simulink model "Q_3_2_a"  (R2023b)
settings: Solver=VariableStepAuto  StartTime=0.0  StopTime=400e-3  MaxStep=tstepMax  RelTol=1e-3
values from neighbouring files (symbols this model uses):
  v_in = 15*sqrt(2)    [Q3_2.m]    (also in thyristor.m = 20)
libraries: spsDiodeLib x6, spsSeriesRLCBranchLib x4, spsACVoltageSourceLib x3, spsCurrentMeasurementLib x2, spsVoltageMeasurementLib x2, spsControlledCurrentSourceLib x1, spsControlledVoltageSourceLib x1, spspowerguiLib x1
settings Model: Creator=abdulkadir  LastModifiedBy=abdulkadir
settings DataIOCC: ReturnWorkspaceOutputs=off

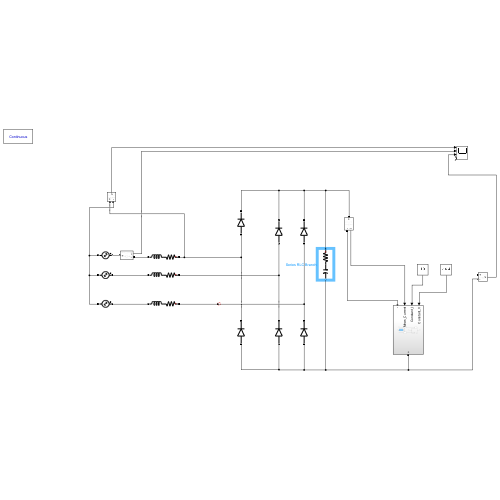
[thumbnail: Simulink's stored preview of the top-level diagram]
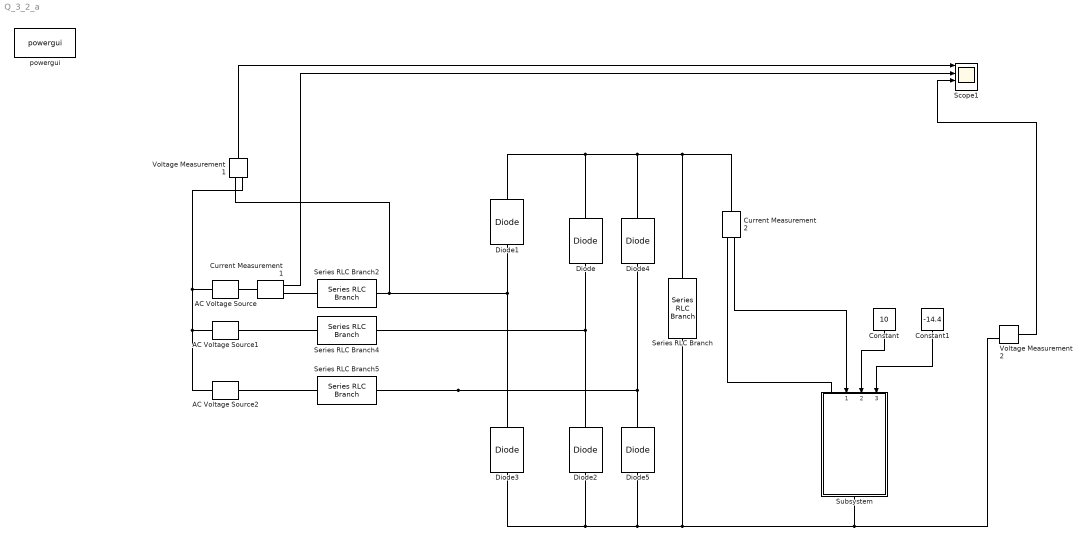
== system Q_3_2_a ==
  AC Voltage Source : spsACVoltageSourceLib/AC Voltage Source  Amplitude=v_in  Phase=0  Frequency=50  SampleTime=0  Measurements=None  BusType=swing  Pref=10e3  Qref=0  Qmin=-inf  Qmax=+inf
  AC Voltage Source1 : spsACVoltageSourceLib/AC Voltage Source  Amplitude=v_in  Phase=120  Frequency=50  SampleTime=0  Measurements=None  BusType=swing  Pref=10e3  Qref=0  Qmin=-inf  Qmax=+inf
  AC Voltage Source2 : spsACVoltageSourceLib/AC Voltage Source  Amplitude=v_in  Phase=240  Frequency=50  SampleTime=0  Measurements=None  BusType=swing  Pref=10e3  Qref=0  Qmin=-inf  Qmax=+inf
  Constant : Constant  Value=10
  Constant1 : Constant  Value=-14.4
  Current Measurement1 : spsCurrentMeasurementLib/Current Measurement  PhasorSimulation=off  OutputType=Complex  PSBequivalent=0
  Current Measurement2 : spsCurrentMeasurementLib/Current Measurement  PhasorSimulation=off  OutputType=Complex  PSBequivalent=0
  Diode{,1..5} (6 alike) : spsDiodeLib/Diode  Ron=0  Lon=0  Vf=0  IC=0  UseSnubber=0  Rs=0  Cs=0  Measurements=off
  Scope1 : Scope  NumInputPorts=4
  Series RLC Branch : spsSeriesRLCBranchLib/Series RLC Branch  LConnTagsString=__new0  RConnTagsString=__new0  BranchType=RC  Resistance=1e-3  Inductance=1e-3  SetiL0=off  InitialCurrent=0  Capacitance=470e-6  Setx0=off  InitialVoltage=0  Measurements=None
  Series RLC Branch2 : spsSeriesRLCBranchLib/Series RLC Branch  LConnTagsString=__new0  RConnTagsString=__new0  BranchType=RL  Resistance=0.05  Inductance=0.28e-3  SetiL0=off  InitialCurrent=0  Capacitance=470e-6  Setx0=off  InitialVoltage=0  Measurements=None
  Series RLC Branch4 : spsSeriesRLCBranchLib/Series RLC Branch  LConnTagsString=__new0  RConnTagsString=__new0  BranchType=RL  Resistance=0.1  Inductance=0.28e-3  SetiL0=off  InitialCurrent=0  Capacitance=470e-6  Setx0=off  InitialVoltage=0  Measurements=None
  Series RLC Branch5 : spsSeriesRLCBranchLib/Series RLC Branch  LConnTagsString=__new0  RConnTagsString=__new0  BranchType=RL  Resistance=0.1  Inductance=0.28e-3  SetiL0=off  InitialCurrent=0  Capacitance=470e-6  Setx0=off  InitialVoltage=0  Measurements=None
  Subsystem : Subsystem
      settings: PortSchema="{\"entries\":[{\"content\":{\"sides\":[{\"content\":{\"connectorIds\":[\"LConn1\",\"In1\",\"In2\",\"In3\"]},\"type\":\"ConnectorPlacement.EquallySpacedRectSide\",\"uuid\":\"feaae4e9-bb6a-4e16-aae7-51a0d38361ce\"},{\"content\":{\"connectorIds\":[\"RConn1\"],\"side\":\"RIGHT\"},\"type\":\"ConnectorPlacement.EquallySpacedRectSide\",\"uuid\":\"0242307e-3fb3-4380-a5a2-342063310801\"},{\"content\":{\"side\":\"TOP\"},\"type\":\"ConnectorPlacement.EquallySpacedRectSide\",\"uuid\":\"eff0ed2a-871e-41c2-ba24-befc3dd8f64b\"}]},\"type\":\"ConnectorPlacement.EquallySpacedConnector\",\"uuid\":\"58606344-83d6-409b-9606-3c46dbcf5736\"}],\"packageUris\":[\"http://schema.mathworks.com/mf0/Connector/R2020b\"],\"version\":\"1.0\"}"
  Voltage Measurement1 : spsVoltageMeasurementLib/Voltage Measurement  PhasorSimulation=off  OutputType=Complex  PSBequivalent=0
  Voltage Measurement2 : spsVoltageMeasurementLib/Voltage Measurement  PhasorSimulation=off  OutputType=Complex  PSBequivalent=0
  powergui : spspowerguiLib/powergui  Priority=1  SimulationMode=Continuous  SampleTime=0.1e-3  frequency=60  Iterations=50  frequencyindice=50  Pbase=100e6  ErrMax=1e-4  UnitsV=kV  UnitsW=MW  buscounter=0  FunctionMessages=off  echomessages=off  EnableUseOfTLC=off  CurrentSourceSwitches=off  DisableSnubberDevices=off  DisableRonSwitches=off  DisableVfSwitches=off  DisplayEquations=off  AutomaticDiscreteSolvers=off  SolverType=Tustin/Backward Euler (TBE)  Interpol=off  ExternalGateDelay=off  methode=off  Ts=100  x0status=blocks  SPID=on  SwTol=0  HookPort=off  NonlinearTolerance=1e-4  nMaxIteration=100  ContinueOnMaxIteration=off  RestoreLinks=warning  ResistiveCurrentMeasurement=off  Frange=[0:2:500]  Ylog=off  Xlog=on  ShowGrid=off  save=off  variable=ZData  structure=0  ZoomFFT=off  StartTime=0.0  cycles=1  DisplayStyle=1  fundamental=60  FreqAxis=off  MaxFrequency=1000  frequencyindicesteady=1  RmsSteady=1  display=off
  wires:
  Current Measurement1/1 -> Scope1/2
  Voltage Measurement2/1 -> Scope1/3
  Voltage Measurement1/1 -> Scope1/1
  Current Measurement2/1 -> Subsystem/1(Meas_Current)
  Constant/1 -> Subsystem/2(Constant_I)
  Constant1/1 -> Subsystem/3(Constant_V)
  connections:
  Series RLC Branch/LConn1 -- Diode4/RConn1 -- Diode1/RConn1 -- Diode/RConn1 -- Current Measurement2/LConn1
  Series RLC Branch/RConn1 -- Subsystem/RConn1 -- Voltage Measurement2/LConn2 -- Diode5/LConn1 -- Diode3/LConn1 -- Diode2/LConn1
  Current Measurement1/LConn1 -- AC Voltage Source/RConn1
  Series RLC Branch2/LConn1 -- Diode1/LConn1 -- Diode3/RConn1 -- Voltage Measurement1/LConn1
  Current Measurement1/RConn1 -- Series RLC Branch2/RConn1
  Series RLC Branch4/RConn1 -- AC Voltage Source1/RConn1
  Series RLC Branch5/RConn1 -- AC Voltage Source2/RConn1
  Diode2/RConn1 -- Series RLC Branch4/LConn1 -- Diode/LConn1
  Voltage Measurement1/LConn2 -- AC Voltage Source/LConn1 -- AC Voltage Source2/LConn1 -- AC Voltage Source1/LConn1
  Diode5/RConn1 -- Series RLC Branch5/LConn1 -- Diode4/LConn1
  Subsystem/LConn1 -- Current Measurement2/RConn1

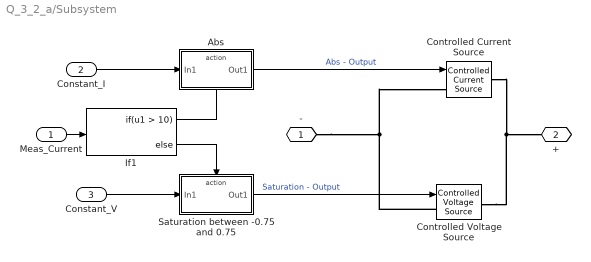
== system Q_3_2_a/Subsystem ==
  Meas_Current : Inport
  Constant_I : Inport  Port=2
  Constant_V : Inport  Port=3
  Abs : Subsystem  TreatAsAtomicUnit=on
  Controlled Current Source : spsControlledCurrentSourceLib/Controlled Current Source  Initialize=on  Source_Type=DC  Amplitude=10  Phase=0  Frequency=0  Measurements=None
  Controlled Voltage Source : spsControlledVoltageSourceLib/Controlled Voltage Source  Initialize=on  Source_Type=DC  Amplitude=14.4  Phase=0  Frequency=0  Measurements=None
  If1 : If  IfExpression=u1 > 10
  Saturation between -0.75 and 0.75 : Subsystem  TreatAsAtomicUnit=on
  - : PMIOPort  Side=Left
  + : PMIOPort  Port=2  Side=Right
  wires:
  If1/2 -> Saturation between -0.75 and 0.75/Action
  Constant_I/1 -> Abs/1(In1)
  Constant_V/1 -> Saturation between -0.75 and 0.75/1(In1)
  If1/1 -> Abs/Action
  Saturation between -0.75 and 0.75/1(Out1) -> Controlled Voltage Source/1  "Saturation - Output"
  Abs/1(Out1) -> Controlled Current Source/1  "Abs - Output"
  Meas_Current/1 -> If1/1
  connections:
  Controlled Voltage Source/LConn1 -- -/RConn1 -- Controlled Current Source/LConn1
  Controlled Current Source/RConn1 -- Controlled Voltage Source/RConn1 -- +/RConn1

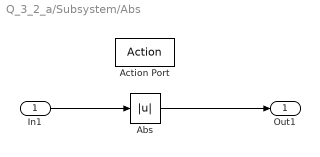
== system Q_3_2_a/Subsystem/Abs ==
  In1 : Inport
  Action Port : ActionPort  ActionPortLabel=if(u1 > 10)
  Abs : Abs  OutDataTypeStr=double
  Out1 : Outport
  wires:
  In1/1 -> Abs/1
  Abs/1 -> Out1/1

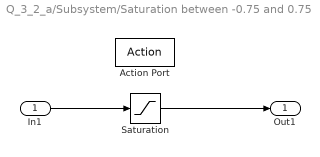
== system Q_3_2_a/Subsystem/Saturation between -0.75 and 0.75 ==
  In1 : Inport
  Action Port : ActionPort  ActionPortLabel=else
  Saturation : Saturate  UpperLimit=0.75  LowerLimit=-0.75
  Out1 : Outport
  wires:
  In1/1 -> Saturation/1
  Saturation/1 -> Out1/1
